simulink library "DC_GRIDSIM_LIB"  (R2022b)
settings: Solver=VariableStepAuto  StartTime=0.0  StopTime=10.0  RelTol=1e-3
undefined symbols (not defined in the file): Allday_timevector, DiscIntNeverNeededParam, High, Household1_Autumnallday, Household1_Springallday, Household1_Summerallday, Household1_Winterallday, Household9_Autumnallday, Household9_Springallday, Household9_Summerallday, Household9_Winterallday, Low, MV, Shift
libraries: fl_lib x66, nesl_utility x33, simulink x8, ee_lib x4
(part 1 of 2)
settings Model: Creator=cfn2169  LastModifiedBy=cfn2169

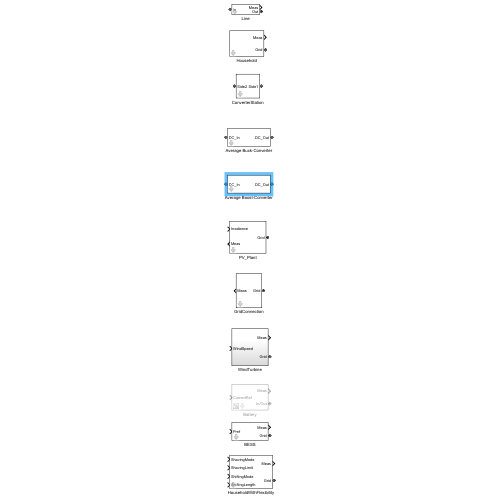
[thumbnail: Simulink's stored preview of the top-level diagram]
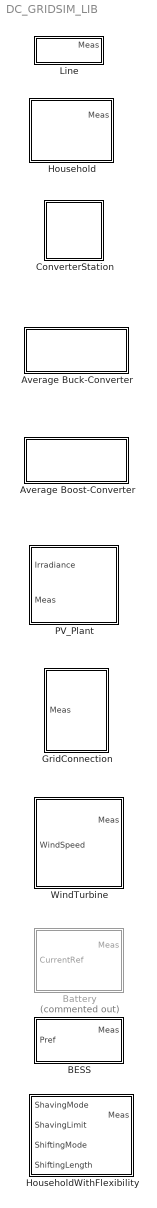
== system DC_GRIDSIM_LIB ==
  Average Boost-Converter : Subsystem  mask{C=1000, D=0.5}
      mask prompts: C "Input/Output Capacities in uF"; D "Duty Cycle"
  Average Buck-Converter : Subsystem  mask{C=1000, D=0.5}
      mask prompts: C "Input/Ouput Capacities in uF"; D "Duty Cycle"
  BESS : Subsystem  mask{V_Bat=380, Qbat=10000, SOC_init=0.5, SOC_min=0.1, SOC_max=0.9, P_max=10000}
      mask prompts: V_Bat "Nominal voltage of battery in V"; Qbat "Battery capacity in Ah"; SOC_init "Initial SOC"; SOC_min "Lower limit for SOC"; SOC_max "Upper limit for SOC"; P_max "Maximum charging/discharging power in W"
  Battery : Subsystem  Commented=on  mask{SOC_Init=0.5, Npar=5, Nser=13, Efull=4.15, Qrat=1.0, Irat=0.2, Eexp=3.7, Qexp=0.85, Enom=3.63, Qnom=0.92, Rint=0.09}
      mask prompts: SOC_Init "Initial SOC"; Npar "Number of cells in parallel"; Nser "Number of cells in series"; Efull "Fully charged voltage in V"; Qrat "Rated capacity in Ah"; Irat "Rated current in A"; Eexp "Voltage at end of exponential zone in V"; Qexp "Charge at end of exponential zone in Ah"; Enom "Voltage at end of nominal zone in V"; Qnom "Charge at end of nominal zone in Ah"; Rint "Internal resistance in Ohm"
      mask DialogControl ParameterGroupVar_1 Prompt: Stack Parameters
      mask DialogControl DescTextVar_1 Prompt: This section defines general parameters for the whole battery. The numbers of connected cells define the overall battery voltage as Vbat = Ecell*Nser and the battery capacity as Qbat = Qcell*Npar.
      mask DialogControl ParameterGroupVar_2 Prompt: Cell Parameters
      mask DialogControl DescTextVar_2 Prompt: This section defines the cell parameters for the battery. They can be found in the datasheet or can be taken from typical charging curves.
  ConverterStation : Subsystem  mask{V_Ref=380}
      mask prompts: V_Ref "Nominal voltage of secondary side"
      mask DialogControl DescTextVar Prompt: Model of a MVDC/LVDC converter station
  GridConnection : Subsystem  mask{MV_Ref=10000}
      mask prompts: MV_Ref "MV voltage reference"
  Household : Subsystem  mask{ProfileSpring=Household1_Springallday, ProfileSummer=Household1_Summerallday, ProfileAutumn=Household1_Autumnallday, ProfileWinter=Household1_Winterallday, Timevector=Allday_timevector, k=1, VnomLoad=380}
      mask prompts: ProfileSpring "Load profile for spring"; ProfileSummer "Load profile for summer"; ProfileAutumn "Load profile for autumn"; ProfileWinter "Load profile for winter"; Timevector "Corresponding timevector"; k "Scaling factor"; VnomLoad "Nominal voltage load"
      mask DialogControl DescTextVar Prompt: Profile-based load model for households
  HouseholdWithFlexibility : Subsystem  mask{Profile_spring=Household9_Springallday, Profile_summer=Household9_Summerallday, Profile_autumn=Household9_Autumnallday, Profile_winter=Household9_Winterallday, Timevector=Allday_timevector, k=1, Vload=380, Base=500, flxQuota=0.5}
      mask prompts: Profile_spring "Load profile for spring"; Profile_summer "Load profile for summer"; Profile_autumn "Load profile for autumn"; Profile_winter "Load profile for winter"; Timevector "Corresponding timevector"; k "Scaling factor"; Vload "Nominal voltage load in V"; Base "Base load in W"; flxQuota "Quota of flexible load"
  Line : Subsystem  mask{rho=1.68e-8, l=1.0, A=240e-6}
      mask prompts: rho "Specific resistivity in Ohm*m"; l "Length in m"; A "Cross sectional area in m^2"
      mask DialogControl DescTextVar Prompt: Resistive line model for two-wired DC systems
  PV_Plant : Subsystem  mask{eta_pv=0.2, area_pv=1000}
      mask prompts: eta_pv "Efficiency of PV modules"; area_pv "Effective area of PV modules in m^2"
      settings: PortSchema="{\"entries\":[{\"content\":{\"sides\":[{\"content\":{\"connectorIds\":[\"LConn1\"]},\"type\":\"ConnectorPlacement.EquallySpacedRectSide\",\"uuid\":\"e7d30e91-d877-4849-85d5-5068117b5a73\"},{\"content\":{\"connectorIds\":[\"In1\",\"Out1\"],\"side\":\"RIGHT\"},\"type\":\"ConnectorPlacement.EquallySpacedRectSide\",\"uuid\":\"aff2ec47-1e97-401e-aec0-02d86814fbc3\"},{\"content\":{\"connectorIds\":[],\"side\":\"TOP\"},\"type\":\"ConnectorPlacement.EquallySpacedRectSide\",\"uuid\":\"0abfbb66-97f7-400f-9c84-fe1e10d1a17f\"}]},\"type\":\"ConnectorPlacement.EquallySpacedConnector\",\"uuid\":\"740b86aa-7ace-499a-bee9-62f02e790000\"}],\"packageUris\":[\"http://schema.mathworks.com/mf0/Connector/R2020b\"],\"version\":\"1.0\"}"
  WindTurbine : Subsystem

== system DC_GRIDSIM_LIB/Average Boost-Converter ==
  PS Constant7 : fl_lib/Physical Signals/Sources/PS Constant  constant=D
  Resistor12 : fl_lib/Electrical/Electrical Elements/Resistor  R=1e6 Ohm  i_specify=off  i_priority=None  i=0 A  i_nominal_specify=off  i_nominal_unit=A  i_nominal_value=1  v_specify=off  v_priority=None  v=0 V  v_nominal_specify=off  v_nominal_unit=V  v_nominal_value=1
  Resistor39 : fl_lib/Electrical/Electrical Elements/Resistor  R=1e6 Ohm  i_specify=off  i_priority=None  i=0 A  i_nominal_specify=off  i_nominal_unit=A  i_nominal_value=1  v_specify=off  v_priority=None  v=0 V  v_nominal_specify=off  v_nominal_unit=V  v_nominal_value=1
  Simscape Bus1 : SimscapeBus  HierarchyStrings=High;Low
  Simscape Bus2 : SimscapeBus  HierarchyStrings=High;Low
  Subsystem5 : Subsystem
  DC_In : PMIOPort  Side=Left
  DC_Out : PMIOPort  Port=2  Side=Right
  connections:
  Resistor12/LConn1 -- Resistor39/RConn1 -- Simscape Bus1/LConn1 -- Subsystem5/RConn1
  Simscape Bus1/LConn2 -- Subsystem5/RConn2 -- Resistor12/RConn1
  Simscape Bus2/LConn2 -- Subsystem5/LConn3 -- Resistor39/LConn1
  Simscape Bus2/RConn1 -- DC_In/RConn1
  Simscape Bus1/RConn1 -- DC_Out/RConn1
  PS Constant7/RConn1 -- Subsystem5/LConn1
  Simscape Bus2/LConn1 -- Subsystem5/LConn2

== system DC_GRIDSIM_LIB/Average Buck-Converter ==
  PS Constant7 : fl_lib/Physical Signals/Sources/PS Constant  constant=D
  Resistor12 : fl_lib/Electrical/Electrical Elements/Resistor  R=1e6 Ohm  i_specify=off  i_priority=None  i=0 A  i_nominal_specify=off  i_nominal_unit=A  i_nominal_value=1  v_specify=off  v_priority=None  v=0 V  v_nominal_specify=off  v_nominal_unit=V  v_nominal_value=1
  Resistor39 : fl_lib/Electrical/Electrical Elements/Resistor  R=1e6 Ohm  i_specify=off  i_priority=None  i=0 A  i_nominal_specify=off  i_nominal_unit=A  i_nominal_value=1  v_specify=off  v_priority=None  v=0 V  v_nominal_specify=off  v_nominal_unit=V  v_nominal_value=1
  Simscape Bus1 : SimscapeBus  HierarchyStrings=High;Low
  Simscape Bus2 : SimscapeBus  HierarchyStrings=High;Low
  Subsystem5 : Subsystem
  DC_In : PMIOPort  Side=Left
  DC_Out : PMIOPort  Port=2  Side=Right
  connections:
  Subsystem5/RConn2 -- Resistor12/RConn1 -- Simscape Bus1/LConn2
  Resistor39/LConn1 -- Subsystem5/LConn3 -- Simscape Bus2/LConn2
  Resistor12/LConn1 -- Resistor39/RConn1 -- Simscape Bus1/LConn1 -- Subsystem5/RConn1
  Simscape Bus2/RConn1 -- DC_In/RConn1
  Subsystem5/LConn2 -- Simscape Bus2/LConn1
  Simscape Bus1/RConn1 -- DC_Out/RConn1
  PS Constant7/RConn1 -- Subsystem5/LConn1

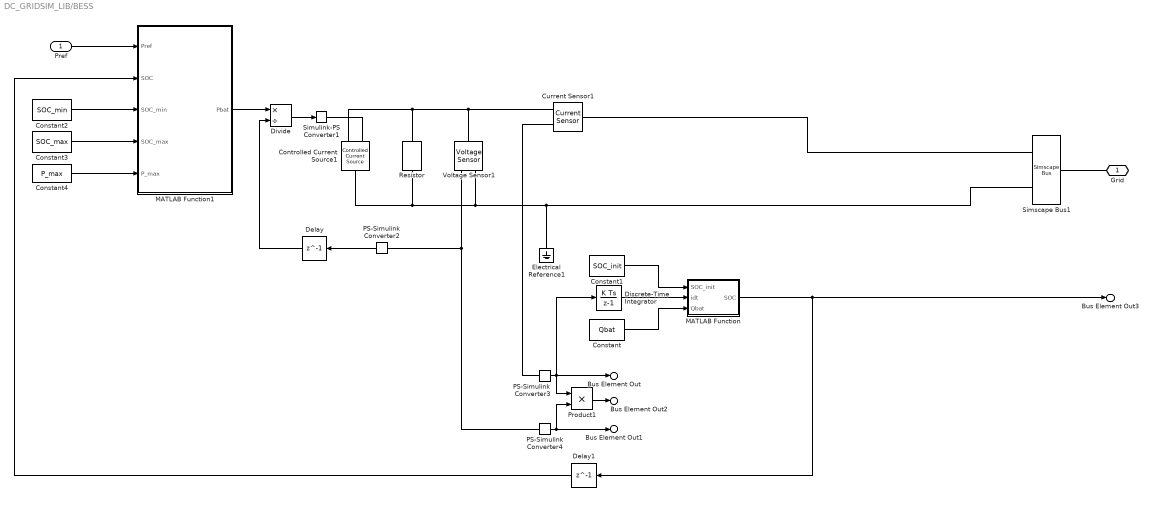
== system DC_GRIDSIM_LIB/BESS ==
  Pref : Inport
  Constant : Constant  Value=Qbat
  Constant1 : Constant  Value=SOC_init
  Constant2 : Constant  Value=SOC_min
  Constant3 : Constant  Value=SOC_max
  Constant4 : Constant  Value=P_max
  Controlled Current Source1 : fl_lib/Electrical/Electrical Sources/Controlled Current Source
  Current Sensor1 : fl_lib/Electrical/Electrical Sensors/Current Sensor
  Delay : Delay  DelayLength=1  InitialCondition=V_Bat
  Delay1 : Delay  DelayLength=1  InitialCondition=SOC_init
  Discrete-Time Integrator : DiscreteIntegrator  SampleTime=-1  ICPrevOutput=DiscIntNeverNeededParam  ICPrevScaledInput=DiscIntNeverNeededParam
  Divide : Product  Inputs=*/
  Electrical Reference1 : fl_lib/Electrical/Electrical Elements/Electrical Reference
  MATLAB Function : MATLAB Function  TreatAsAtomicUnit=on
  MATLAB Function1 : MATLAB Function  TreatAsAtomicUnit=on
  PS-Simulink Converter2 : nesl_utility/PS-Simulink Converter  PhysicalDomain=network_engine_domain  SubClassName=ps_output  LeftPortType=input  RightPortType=output  PseudoPeriodic=off  Frequencies=[]  VectorFormat=inherit  Unit=inherit  AffineConversion=off
  PS-Simulink Converter3 : nesl_utility/PS-Simulink Converter  PhysicalDomain=network_engine_domain  SubClassName=ps_output  LeftPortType=input  RightPortType=output  PseudoPeriodic=off  Frequencies=[]  VectorFormat=inherit  Unit=inherit  AffineConversion=off
  PS-Simulink Converter4 : nesl_utility/PS-Simulink Converter  PhysicalDomain=network_engine_domain  SubClassName=ps_output  LeftPortType=input  RightPortType=output  PseudoPeriodic=off  Frequencies=[]  VectorFormat=inherit  Unit=inherit  AffineConversion=off
  Product1 : Product
  Resistor : fl_lib/Electrical/Electrical Elements/Resistor  R=1e9 Ohm  i_specify=off  i_priority=None  i=0 A  i_nominal_specify=off  i_nominal_unit=A  i_nominal_value=1  v_specify=off  v_priority=None  v=0 V  v_nominal_specify=off  v_nominal_unit=V  v_nominal_value=1
  Simscape Bus1 : SimscapeBus  HierarchyStrings=High;Low
  Simulink-PS Converter1 : nesl_utility/Simulink-PS Converter  PhysicalDomain=network_engine_domain  SubClassName=ps_input  LeftPortType=input  RightPortType=output  PseudoPeriodic=off  Frequencies=[]  NoiseDistribution=none  NoiseParameters=[]  Unit=1  AffineConversion=off  FilteringAndDerivatives=provide  SimscapeFilterOrder=1  InputFilterTimeConstant=0.001  UdotUserProvided=0
  Voltage Sensor1 : fl_lib/Electrical/Electrical Sensors/Voltage Sensor
  Grid : PMIOPort  Side=Right
  Bus Element Out : Outport  PortName=Meas  Element=Current
  Bus Element Out1 : Outport  PortName=Meas  Element=Voltage
  Bus Element Out2 : Outport  PortName=Meas  Element=Power
  Bus Element Out3 : Outport  PortName=Meas  Element=SOC
  wires:
  Product1/1 -> Bus Element Out2/1
  MATLAB Function1/1(Pbat) -> Divide/1
  PS-Simulink Converter3/1 -> Discrete-Time Integrator/1, Product1/1, Bus Element Out/1
  Delay/1 -> Divide/2
  Divide/1 -> Simulink-PS Converter1/1
  PS-Simulink Converter4/1 -> Product1/2, Bus Element Out1/1
  PS-Simulink Converter2/1 -> Delay/1
  Discrete-Time Integrator/1 -> MATLAB Function/2(idt)
  Constant/1 -> MATLAB Function/3(Qbat)
  Constant1/1 -> MATLAB Function/1(SOC_init)
  MATLAB Function/1(SOC) -> Bus Element Out3/1, Delay1/1
  Pref/1 -> MATLAB Function1/1(Pref)
  Delay1/1 -> MATLAB Function1/2(SOC)
  Constant2/1 -> MATLAB Function1/3(SOC_min)
  Constant3/1 -> MATLAB Function1/4(SOC_max)
  Constant4/1 -> MATLAB Function1/5(P_max)
  connections:
  Voltage Sensor1/LConn1 -- Resistor/LConn1 -- Controlled Current Source1/RConn2 -- Current Sensor1/RConn2
  PS-Simulink Converter2/LConn1 -- PS-Simulink Converter4/LConn1 -- Voltage Sensor1/RConn1
  Simscape Bus1/LConn1 -- Current Sensor1/LConn1
  PS-Simulink Converter3/LConn1 -- Current Sensor1/RConn1
  Simulink-PS Converter1/RConn1 -- Controlled Current Source1/RConn1
  Grid/RConn1 -- Simscape Bus1/RConn1
  Resistor/RConn1 -- Controlled Current Source1/LConn1 -- Voltage Sensor1/RConn2 -- Simscape Bus1/LConn2 -- Electrical Reference1/LConn1

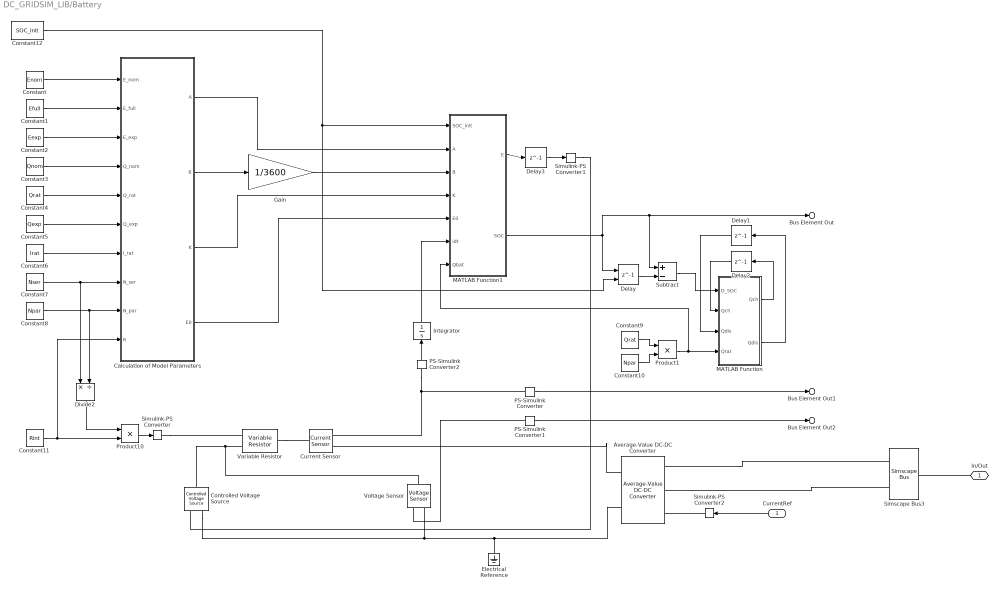
== system DC_GRIDSIM_LIB/Battery ==
  CurrentRef : Inport
  Average-Value DC-DC Converter : ee_lib/Semiconductors & Converters/Converters/Average-Value DC-DC Converter  control_option=ee.enum.converters.controlinput.current  converter_type=ee.enum.converters.dcdctype.buck  efficiency_option=ee.enum.converters.efficiency.constant  efficiency_fixed=100  i_vec=[0, 2, 5] A  efficiency_vec=[90, 95, 98]
      settings: InternalSimscapePortConfiguration="{\"Bottom\":[],\"Left\":[{\"id\":\"Iref\",\"label\":\"Iref\",\"type\":\"input\"},{\"id\":\"p1\",\"label\":\"1+\",\"type\":\"foundation.electrical.electrical\"},{\"id\":\"n1\",\"label\":\"1-\",\"type\":\"foundation.electrical.electrical\"}],\"Right\":[{\"id\":\"p2\",\"label\":\"2+\",\"type\":\"foundation.electrical.electrical\"},{\"id\":\"n2\",\"label\":\"2-\",\"type\":\"foundation.electrical.electrical\"}],\"Top\":[]}"
  Calculation of Model Parameters : Subsystem
  Constant : Constant  Value=Enom
  Constant1 : Constant  Value=Efull
  Constant10 : Constant  Value=Npar
  Constant11 : Constant  Value=Rint
  Constant12 : Constant  Value=SOC_Init
  Constant2 : Constant  Value=Eexp
  Constant3 : Constant  Value=Qnom
  Constant4 : Constant  Value=Qrat
  Constant5 : Constant  Value=Qexp
  Constant6 : Constant  Value=Irat
  Constant7 : Constant  Value=Nser
  Constant8 : Constant  Value=Npar
  Constant9 : Constant  Value=Qrat
  Controlled Voltage Source : fl_lib/Electrical/Electrical Sources/Controlled Voltage Source
  Current Sensor : fl_lib/Electrical/Electrical Sensors/Current Sensor
  Delay : Delay  DelayLength=1  InitialConditionSource=Input port
      settings: InputPortMap=u0,p4
  Delay1 : Delay  DelayLength=1
  Delay2 : Delay  DelayLength=1
  Delay3 : Delay  DelayLength=1  InitialCondition=Enom*Nser
  Divide2 : Product  Inputs=*/
  Electrical Reference : fl_lib/Electrical/Electrical Elements/Electrical Reference
  Gain : Gain  Gain=1/3600
  Integrator : Integrator
  MATLAB Function : MATLAB Function  TreatAsAtomicUnit=on
  MATLAB Function1 : MATLAB Function  TreatAsAtomicUnit=on
  PS-Simulink Converter : nesl_utility/PS-Simulink Converter  PhysicalDomain=network_engine_domain  SubClassName=ps_output  LeftPortType=input  RightPortType=output  PseudoPeriodic=off  Frequencies=[]  VectorFormat=1-D array  Unit=inherit  AffineConversion=off
  PS-Simulink Converter1 : nesl_utility/PS-Simulink Converter  PhysicalDomain=network_engine_domain  SubClassName=ps_output  LeftPortType=input  RightPortType=output  PseudoPeriodic=off  Frequencies=[]  VectorFormat=1-D array  Unit=inherit  AffineConversion=off
  PS-Simulink Converter2 : nesl_utility/PS-Simulink Converter  PhysicalDomain=network_engine_domain  SubClassName=ps_output  LeftPortType=input  RightPortType=output  PseudoPeriodic=off  Frequencies=[]  VectorFormat=1-D array  Unit=inherit  AffineConversion=off
  Product1 : Product
  Product10 : Product
  Simscape Bus3 : SimscapeBus  HierarchyStrings=Low;High
  Simulink-PS Converter : nesl_utility/Simulink-PS Converter  PhysicalDomain=network_engine_domain  SubClassName=ps_input  LeftPortType=input  RightPortType=output  PseudoPeriodic=off  Frequencies=[]  NoiseDistribution=none  NoiseParameters=[]  Unit=1  AffineConversion=off  FilteringAndDerivatives=provide  SimscapeFilterOrder=1  InputFilterTimeConstant=0.001  UdotUserProvided=0
  Simulink-PS Converter1 : nesl_utility/Simulink-PS Converter  PhysicalDomain=network_engine_domain  SubClassName=ps_input  LeftPortType=input  RightPortType=output  PseudoPeriodic=off  Frequencies=[]  NoiseDistribution=none  NoiseParameters=[]  Unit=1  AffineConversion=off  FilteringAndDerivatives=provide  SimscapeFilterOrder=1  InputFilterTimeConstant=0.001  UdotUserProvided=0
  Simulink-PS Converter2 : nesl_utility/Simulink-PS Converter  PhysicalDomain=network_engine_domain  SubClassName=ps_input  LeftPortType=input  RightPortType=output  PseudoPeriodic=off  Frequencies=[]  NoiseDistribution=none  NoiseParameters=[]  Unit=1  AffineConversion=off  FilteringAndDerivatives=provide  SimscapeFilterOrder=1  InputFilterTimeConstant=0.001  UdotUserProvided=0
  Subtract : Sum  Inputs=+-
  Variable Resistor : fl_lib/Electrical/Electrical Elements/Variable Resistor  Rmin=0 Ohm  i_specify=off  i_priority=None  i=0 A  i_nominal_specify=off  i_nominal_unit=A  i_nominal_value=1  v_specify=off  v_priority=None  v=0 V  v_nominal_specify=off  v_nominal_unit=V  v_nominal_value=1
  Voltage Sensor : fl_lib/Electrical/Electrical Sensors/Voltage Sensor
  In/Out : PMIOPort  Side=Right
  Bus Element Out : Outport  PortName=Meas  Element=SOC
  Bus Element Out1 : Outport  PortName=Meas  Element=Current
  Bus Element Out2 : Outport  PortName=Meas  Element=Voltage
  wires:
  Integrator/1 -> MATLAB Function1/6(idt)
  Constant7/1 -> Calculation of Model Parameters/8(N_ser), Divide2/1
  MATLAB Function/2(Qdis) -> Delay1/1
  PS-Simulink Converter2/1 -> Integrator/1
  Constant8/1 -> Calculation of Model Parameters/9(N_par), Divide2/2
  Calculation of Model Parameters/3(K) -> MATLAB Function1/4(K)
  Delay2/1 -> MATLAB Function/2("Qch ")
  MATLAB Function/1(Qch) -> Delay2/1
  Constant9/1 -> Product1/1
  PS-Simulink Converter1/1 -> Bus Element Out2/1
  PS-Simulink Converter/1 -> Bus Element Out1/1
  Calculation of Model Parameters/4(E0) -> MATLAB Function1/5(E0)
  Delay1/1 -> MATLAB Function/3("Qdis ")
  Gain/1 -> MATLAB Function1/3(B)
  Calculation of Model Parameters/1(A) -> MATLAB Function1/2(A)
  Constant12/1 -> Delay/2, MATLAB Function1/1(SOC_init)
  Product10/1 -> Simulink-PS Converter/1
  Constant/1 -> Calculation of Model Parameters/1(E_nom)
  Calculation of Model Parameters/2(B) -> Gain/1
  Constant1/1 -> Calculation of Model Parameters/2(E_full)
  Subtract/1 -> MATLAB Function/1(D_SOC)
  Constant6/1 -> Calculation of Model Parameters/7(I_rat)
  Constant10/1 -> Product1/2
  Constant4/1 -> Calculation of Model Parameters/5(Q_rat)
  Constant5/1 -> Calculation of Model Parameters/6(Q_exp)
  Divide2/1 -> Product10/1
  MATLAB Function1/2(SOC) -> Bus Element Out/1, Subtract/1, Delay/1
  Constant11/1 -> Product10/2, Calculation of Model Parameters/10(R)
  Constant3/1 -> Calculation of Model Parameters/4(Q_nom)
  Constant2/1 -> Calculation of Model Parameters/3(E_exp)
  Product1/1 -> MATLAB Function1/7(Qbat), MATLAB Function/4(Qrat)
  Delay/1 -> Subtract/2
  MATLAB Function1/1(E) -> Delay3/1
  Delay3/1 -> Simulink-PS Converter1/1
  CurrentRef/1 -> Simulink-PS Converter2/1
  connections:
  PS-Simulink Converter/LConn1 -- PS-Simulink Converter2/LConn1 -- Current Sensor/RConn1
  Electrical Reference/LConn1 -- Average-Value DC-DC Converter/RConn1 -- Controlled Voltage Source/RConn2 -- Voltage Sensor/RConn2
  Voltage Sensor/LConn1 -- Controlled Voltage Source/LConn1 -- Variable Resistor/LConn2
  Simulink-PS Converter1/RConn1 -- Controlled Voltage Source/RConn1
  Average-Value DC-DC Converter/RConn2 -- Current Sensor/RConn2
  Simulink-PS Converter/RConn1 -- Variable Resistor/LConn1
  Variable Resistor/RConn1 -- Current Sensor/LConn1
  PS-Simulink Converter1/LConn1 -- Voltage Sensor/RConn1
  Simulink-PS Converter2/RConn1 -- Average-Value DC-DC Converter/LConn1
  In/Out/RConn1 -- Simscape Bus3/RConn1
  Simscape Bus3/LConn2 -- Average-Value DC-DC Converter/LConn2
  Simscape Bus3/LConn1 -- Average-Value DC-DC Converter/LConn3

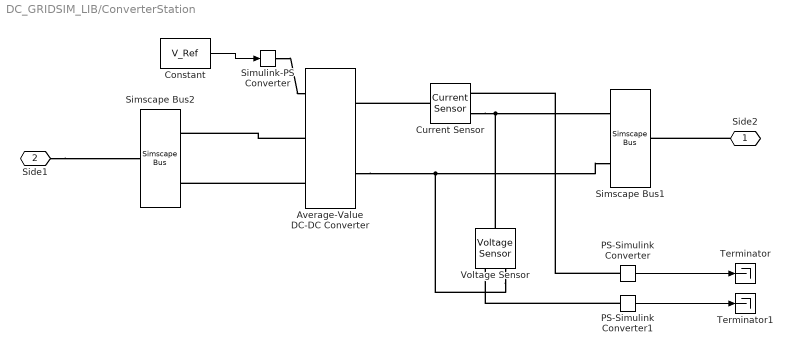
== system DC_GRIDSIM_LIB/ConverterStation ==
  Average-Value DC-DC Converter : ee_lib/Semiconductors & Converters/Converters/Average-Value DC-DC Converter  control_option=ee.enum.converters.controlinput.voltage  converter_type=ee.enum.converters.dcdctype.buck  efficiency_option=ee.enum.converters.efficiency.constant  efficiency_fixed=100  i_vec=[0, 2, 5] A  efficiency_vec=[90, 95, 98]
      settings: InternalSimscapePortConfiguration="{\"Bottom\":[],\"Left\":[{\"id\":\"Vref\",\"label\":\"Vref\",\"type\":\"input\"},{\"id\":\"p1\",\"label\":\"1+\",\"type\":\"foundation.electrical.electrical\"},{\"id\":\"n1\",\"label\":\"1-\",\"type\":\"foundation.electrical.electrical\"}],\"Right\":[{\"id\":\"p2\",\"label\":\"2+\",\"type\":\"foundation.electrical.electrical\"},{\"id\":\"n2\",\"label\":\"2-\",\"type\":\"foundation.electrical.electrical\"}],\"Top\":[]}"
  Constant : Constant  Value=V_Ref
  Current Sensor : fl_lib/Electrical/Electrical Sensors/Current Sensor
  PS-Simulink Converter : nesl_utility/PS-Simulink Converter  PhysicalDomain=network_engine_domain  SubClassName=ps_output  LeftPortType=input  RightPortType=output  PseudoPeriodic=off  Frequencies=[]  VectorFormat=inherit  Unit=inherit  AffineConversion=off
  PS-Simulink Converter1 : nesl_utility/PS-Simulink Converter  PhysicalDomain=network_engine_domain  SubClassName=ps_output  LeftPortType=input  RightPortType=output  PseudoPeriodic=off  Frequencies=[]  VectorFormat=inherit  Unit=inherit  AffineConversion=off
  Simscape Bus1 : SimscapeBus  HierarchyStrings=High;Low
  Simscape Bus2 : SimscapeBus  HierarchyStrings=High;Low
  Simulink-PS Converter : nesl_utility/Simulink-PS Converter  PhysicalDomain=network_engine_domain  SubClassName=ps_input  LeftPortType=input  RightPortType=output  PseudoPeriodic=off  Frequencies=[]  NoiseDistribution=none  NoiseParameters=[]  Unit=1  AffineConversion=off  FilteringAndDerivatives=provide  SimscapeFilterOrder=1  InputFilterTimeConstant=0.001  UdotUserProvided=0
  Terminator : Terminator
  Terminator1 : Terminator
  Voltage Sensor : fl_lib/Electrical/Electrical Sensors/Voltage Sensor
  Side2 : PMIOPort  Side=Left
  Side1 : PMIOPort  Port=2  Side=Right
  wires:
  PS-Simulink Converter/1 -> Terminator/1
  PS-Simulink Converter1/1 -> Terminator1/1
  Constant/1 -> Simulink-PS Converter/1
  connections:
  Voltage Sensor/RConn2 -- Average-Value DC-DC Converter/RConn2 -- Simscape Bus1/LConn2
  Voltage Sensor/LConn1 -- Simscape Bus1/LConn1 -- Current Sensor/RConn2
  Current Sensor/LConn1 -- Average-Value DC-DC Converter/RConn1
  PS-Simulink Converter/LConn1 -- Current Sensor/RConn1
  Average-Value DC-DC Converter/LConn2 -- Simscape Bus2/LConn1
  Average-Value DC-DC Converter/LConn3 -- Simscape Bus2/LConn2
  Simulink-PS Converter/RConn1 -- Average-Value DC-DC Converter/LConn1
  PS-Simulink Converter1/LConn1 -- Voltage Sensor/RConn1
  Side2/RConn1 -- Simscape Bus1/RConn1
  Side1/RConn1 -- Simscape Bus2/RConn1

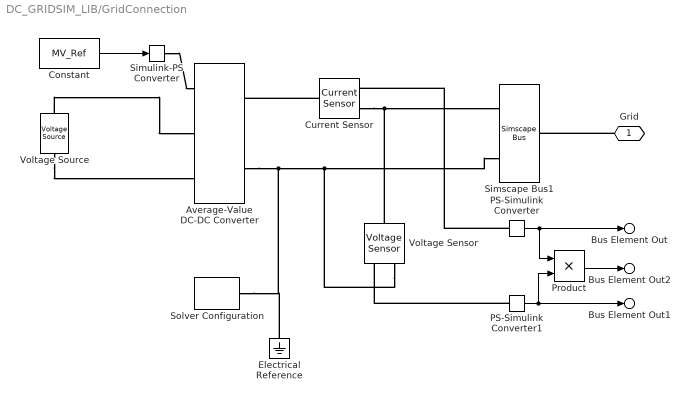
== system DC_GRIDSIM_LIB/GridConnection ==
  Average-Value DC-DC Converter : ee_lib/Semiconductors & Converters/Converters/Average-Value DC-DC Converter  control_option=ee.enum.converters.controlinput.voltage  converter_type=ee.enum.converters.dcdctype.buck  efficiency_option=ee.enum.converters.efficiency.constant  efficiency_fixed=100  i_vec=[0, 2, 5] A  efficiency_vec=[90, 95, 98]
      settings: InternalSimscapePortConfiguration="{\"Bottom\":[],\"Left\":[{\"id\":\"Vref\",\"label\":\"Vref\",\"type\":\"input\"},{\"id\":\"p1\",\"label\":\"1+\",\"type\":\"foundation.electrical.electrical\"},{\"id\":\"n1\",\"label\":\"1-\",\"type\":\"foundation.electrical.electrical\"}],\"Right\":[{\"id\":\"p2\",\"label\":\"2+\",\"type\":\"foundation.electrical.electrical\"},{\"id\":\"n2\",\"label\":\"2-\",\"type\":\"foundation.electrical.electrical\"}],\"Top\":[]}"
  Constant : Constant  Value=MV_Ref
  Current Sensor : fl_lib/Electrical/Electrical Sensors/Current Sensor
  Electrical Reference : fl_lib/Electrical/Electrical Elements/Electrical Reference
  PS-Simulink Converter : nesl_utility/PS-Simulink Converter  PhysicalDomain=network_engine_domain  SubClassName=ps_output  LeftPortType=input  RightPortType=output  PseudoPeriodic=off  Frequencies=[]  VectorFormat=inherit  Unit=inherit  AffineConversion=off
  PS-Simulink Converter1 : nesl_utility/PS-Simulink Converter  PhysicalDomain=network_engine_domain  SubClassName=ps_output  LeftPortType=input  RightPortType=output  PseudoPeriodic=off  Frequencies=[]  VectorFormat=inherit  Unit=inherit  AffineConversion=off
  Product : Product
  Simscape Bus1 : SimscapeBus  HierarchyStrings=High;Low
  Simulink-PS Converter : nesl_utility/Simulink-PS Converter  PhysicalDomain=network_engine_domain  SubClassName=ps_input  LeftPortType=input  RightPortType=output  PseudoPeriodic=off  Frequencies=[]  NoiseDistribution=none  NoiseParameters=[]  Unit=1  AffineConversion=off  FilteringAndDerivatives=provide  SimscapeFilterOrder=1  InputFilterTimeConstant=0.001  UdotUserProvided=0
  Solver Configuration : nesl_utility/Solver Configuration  PhysicalDomain=network_engine_domain  SubClassName=solver  LeftPortType=input  RightPortType=generic  Tones=[]  Harmonics=[]  SimulateNoise=off  Profile=off  UseLocalSampling=off  EnableSwitchedLinearOptims=on  FrequencyDomain=off  UseCCode=off  RelTol=0.001  AbsTol=0.001  MinStep=1e-09  ToWorkspace=off  RevertToSquareIcSolve=off  NumHomotopyIterations=100  PhasorMode=off  PhasorModeNumHarmonics=1  ConsistencySolver=NEWTON_XTOL_AFTER_FTOL  IndexReductionMethod=DerivativeReplacement  DoDC=off  ResidualTolerance=1e-09  ConsistencyTolSource=GLOBAL  ConsistencyAbsTol=0.001  ConsistencyRelTol=0.001  ConsistencyTolFactor=0.001  UseLocalSolver=off  LocalSolverChoice=NE_BACKWARD_EULER_ADVANCER  ResolveIndetEquations=on  FunctionEvalNumThread=1  LocalSolverSampleTime=0.001  DoFixedCost=off  MaxNonlinIter=3  MaxModeIter=2  ComputeImpulses=off  ImpulseIterations=2  LinearAlgebra=auto  LinearAlgebraNumThread=0  EquationFormulation=NE_TIME_EF  DelaysMemoryBudget=1024  AutomaticFiltering=on  FilteringTimeConstant=0.001  PartitionStorageMethod=AS_NEEDED  PartitionMemoryBudget=1024  PartitionMethod=ROBUST
  Voltage Sensor : fl_lib/Electrical/Electrical Sensors/Voltage Sensor
  Voltage Source : ee_lib/Sources/Voltage Source  dc_voltage=10000 V  ac_voltage=0 V  ac_shift=0 rad  ac_frequency=60 Hz  noise_mode=ee.enum.sources.noise.Disabled  PSD=0 V^2/Hz  sample_time=1e-3 s  repeatability=ee.enum.sources.repeatability.NotRepeatable  user_seed=0  auto_seed=3499211588  i_specify=off  i_priority=None  i=0 A  i_nominal_specify=off  i_nominal_unit=A  i_nominal_value=1  v_specify=off  v_priority=None  v=0 V  v_nominal_specify=off  v_nominal_unit=V  v_nominal_value=1
  Grid : PMIOPort  Side=Left
  Bus Element Out : Outport  PortName=Meas  Element=Current
  Bus Element Out1 : Outport  PortName=Meas  Element=Voltage
  Bus Element Out2 : Outport  PortName=Meas  Element=Power
  wires:
  Constant/1 -> Simulink-PS Converter/1
  PS-Simulink Converter/1 -> Product/1, Bus Element Out/1
  PS-Simulink Converter1/1 -> Product/2, Bus Element Out1/1
  Product/1 -> Bus Element Out2/1
  connections:
  Grid/RConn1 -- Simscape Bus1/RConn1
  Voltage Source/LConn1 -- Average-Value DC-DC Converter/LConn2
  Voltage Source/RConn1 -- Average-Value DC-DC Converter/LConn3
  Simulink-PS Converter/RConn1 -- Average-Value DC-DC Converter/LConn1
  Average-Value DC-DC Converter/RConn2 -- Solver Configuration/RConn1 -- Electrical Reference/LConn1 -- Voltage Sensor/RConn2 -- Simscape Bus1/LConn2
  Current Sensor/RConn2 -- Voltage Sensor/LConn1 -- Simscape Bus1/LConn1
  Current Sensor/LConn1 -- Average-Value DC-DC Converter/RConn1
  PS-Simulink Converter1/LConn1 -- Voltage Sensor/RConn1
  PS-Simulink Converter/LConn1 -- Current Sensor/RConn1

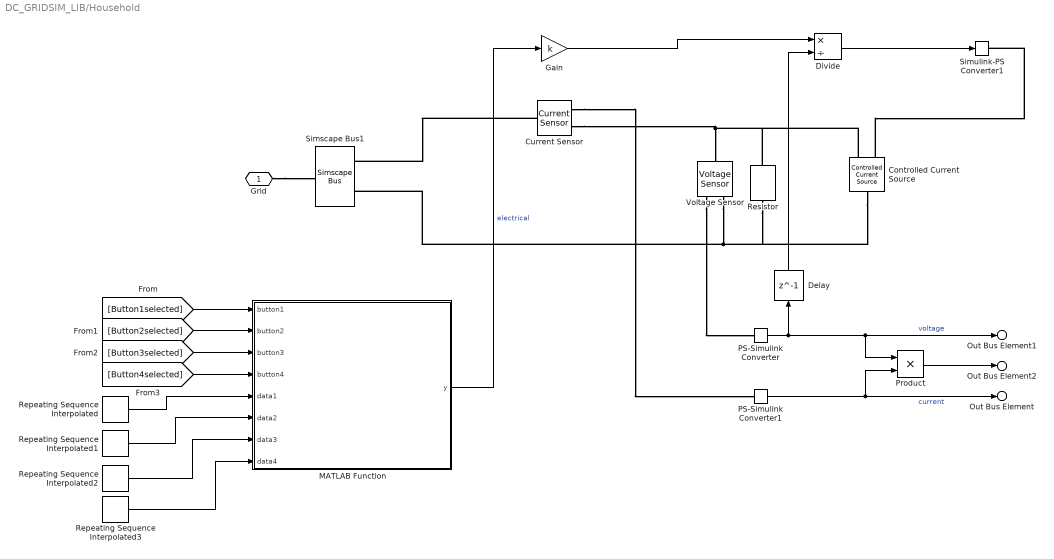
== system DC_GRIDSIM_LIB/Household ==
  Controlled Current Source : fl_lib/Electrical/Electrical Sources/Controlled Current Source
  Current Sensor : fl_lib/Electrical/Electrical Sensors/Current Sensor
  Delay : Delay  DelayLength=1  InitialCondition=VnomLoad
  Divide : Product  Inputs=*/
  Gain : Gain  Gain=k
  MATLAB Function : MATLAB Function  TreatAsAtomicUnit=on
  PS-Simulink Converter : nesl_utility/PS-Simulink Converter  PhysicalDomain=network_engine_domain  SubClassName=ps_output  LeftPortType=input  RightPortType=output  PseudoPeriodic=off  Frequencies=[]  VectorFormat=inherit  Unit=inherit  AffineConversion=off
  PS-Simulink Converter1 : nesl_utility/PS-Simulink Converter  PhysicalDomain=network_engine_domain  SubClassName=ps_output  LeftPortType=input  RightPortType=output  PseudoPeriodic=off  Frequencies=[]  VectorFormat=inherit  Unit=inherit  AffineConversion=off
  Product : Product
  Repeating Sequence Interpolated : simulink/Sources/Repeating Sequence Interpolated  OutValues=ProfileSpring  TimeValues=Timevector  LookUpMeth=Interpolation-Use End Values  tsamp=0.01  OutMin=[]  OutMax=[]  OutDataTypeStr=double  OutputDataTypeScalingMode=double  OutDataType=fixdt(0,8)  OutScaling=2^-10
  Repeating Sequence Interpolated1 : simulink/Sources/Repeating Sequence Interpolated  OutValues=ProfileSummer  TimeValues=Timevector  LookUpMeth=Interpolation-Use End Values  tsamp=0.01  OutMin=[]  OutMax=[]  OutDataTypeStr=double  OutputDataTypeScalingMode=double  OutDataType=fixdt(0,8)  OutScaling=2^-10
  Repeating Sequence Interpolated2 : simulink/Sources/Repeating Sequence Interpolated  OutValues=ProfileAutumn  TimeValues=Timevector  LookUpMeth=Interpolation-Use End Values  tsamp=0.01  OutMin=[]  OutMax=[]  OutDataTypeStr=double  OutputDataTypeScalingMode=double  OutDataType=fixdt(0,8)  OutScaling=2^-10
  Repeating Sequence Interpolated3 : simulink/Sources/Repeating Sequence Interpolated  OutValues=ProfileWinter  TimeValues=Timevector  LookUpMeth=Interpolation-Use End Values  tsamp=0.01  OutMin=[]  OutMax=[]  OutDataTypeStr=double  OutputDataTypeScalingMode=double  OutDataType=fixdt(0,8)  OutScaling=2^-10
  Resistor : fl_lib/Electrical/Electrical Elements/Resistor  R=1e9 Ohm  i_specify=off  i_priority=None  i=0 A  i_nominal_specify=off  i_nominal_unit=A  i_nominal_value=1  v_specify=off  v_priority=None  v=0 V  v_nominal_specify=off  v_nominal_unit=V  v_nominal_value=1
  Simscape Bus1 : SimscapeBus  HierarchyStrings=High;Low
  Simulink-PS Converter1 : nesl_utility/Simulink-PS Converter  PhysicalDomain=network_engine_domain  SubClassName=ps_input  LeftPortType=input  RightPortType=output  PseudoPeriodic=off  Frequencies=[]  NoiseDistribution=none  NoiseParameters=[]  Unit=1  AffineConversion=off  FilteringAndDerivatives=provide  SimscapeFilterOrder=1  InputFilterTimeConstant=0.001  UdotUserProvided=0
  Voltage Sensor : fl_lib/Electrical/Electrical Sensors/Voltage Sensor
  Grid : PMIOPort  Side=Right
  Out Bus Element : Outport  PortName=Meas  Element=Current
  Out Bus Element1 : Outport  PortName=Meas  Element=Voltage
  Out Bus Element2 : Outport  PortName=Meas  Element=Power
  wires:
  MATLAB Function/1(y) -> Gain/1  "electrical"
  PS-Simulink Converter/1 -> Delay/1, Product/1, Out Bus Element1/1  "voltage"
  PS-Simulink Converter1/1 -> Product/2, Out Bus Element/1  "current"
  [Button4selected] -> MATLAB Function/4(button4)
  [Button3selected] -> MATLAB Function/3(button3)
  [Button2selected] -> MATLAB Function/2(button2)
  [Button1selected] -> MATLAB Function/1(button1)
  Repeating Sequence Interpolated/1 -> MATLAB Function/5(data1)
  Repeating Sequence Interpolated1/1 -> MATLAB Function/6(data2)
  Repeating Sequence Interpolated2/1 -> MATLAB Function/7(data3)
  Repeating Sequence Interpolated3/1 -> MATLAB Function/8(data4)
  Product/1 -> Out Bus Element2/1
  Gain/1 -> Divide/1
  Delay/1 -> Divide/2
  Divide/1 -> Simulink-PS Converter1/1
  connections:
  Grid/RConn1 -- Simscape Bus1/RConn1
  Voltage Sensor/RConn2 -- Resistor/RConn1 -- Controlled Current Source/LConn1 -- Simscape Bus1/LConn2
  Voltage Sensor/RConn1 -- PS-Simulink Converter/LConn1
  Current Sensor/RConn1 -- PS-Simulink Converter1/LConn1
  Current Sensor/LConn1 -- Simscape Bus1/LConn1
  Current Sensor/RConn2 -- Resistor/LConn1 -- Controlled Current Source/RConn2 -- Voltage Sensor/LConn1
  Controlled Current Source/RConn1 -- Simulink-PS Converter1/RConn1

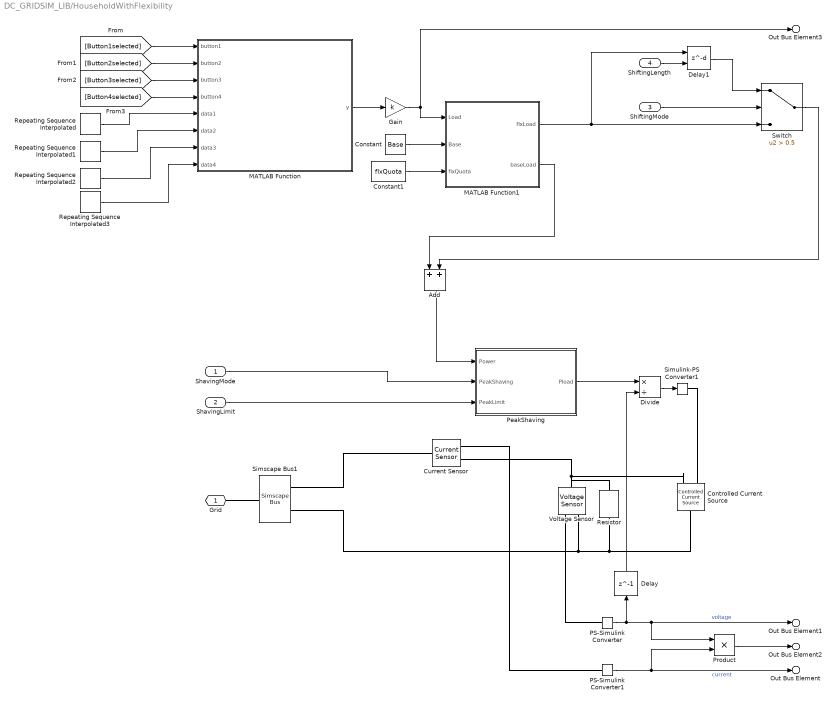
== system DC_GRIDSIM_LIB/HouseholdWithFlexibility ==
  ShavingMode : Inport
  ShavingLimit : Inport  Port=2
  ShiftingMode : Inport  Port=3
  ShiftingLength : Inport  Port=4
  Add : Sum
  Constant : Constant  Value=Base
  Constant1 : Constant  Value=flxQuota
  Controlled Current Source : fl_lib/Electrical/Electrical Sources/Controlled Current Source
  Current Sensor : fl_lib/Electrical/Electrical Sensors/Current Sensor
  Delay : Delay  DelayLength=1  InitialCondition=Vload
  Delay1 : Delay  DelayLengthSource=Input port  DelayLength=Shift  DelayLengthUpperLimit=1000
      settings: InputPortMap=u0,p1
  Divide : Product  Inputs=*/
  Gain : Gain  Gain=k
  MATLAB Function : MATLAB Function  TreatAsAtomicUnit=on
  MATLAB Function1 : MATLAB Function  TreatAsAtomicUnit=on
  PS-Simulink Converter : nesl_utility/PS-Simulink Converter  PhysicalDomain=network_engine_domain  SubClassName=ps_output  LeftPortType=input  RightPortType=output  PseudoPeriodic=off  Frequencies=[]  VectorFormat=inherit  Unit=inherit  AffineConversion=off
  PS-Simulink Converter1 : nesl_utility/PS-Simulink Converter  PhysicalDomain=network_engine_domain  SubClassName=ps_output  LeftPortType=input  RightPortType=output  PseudoPeriodic=off  Frequencies=[]  VectorFormat=inherit  Unit=inherit  AffineConversion=off
  PeakShaving : MATLAB Function  TreatAsAtomicUnit=on
  Product : Product
  Repeating Sequence Interpolated : simulink/Sources/Repeating Sequence Interpolated  OutValues=Profile_spring  TimeValues=Timevector  LookUpMeth=Interpolation-Use End Values  tsamp=0.01  OutMin=[]  OutMax=[]  OutDataTypeStr=double  OutputDataTypeScalingMode=double  OutDataType=fixdt(0,8)  OutScaling=2^-10
  Repeating Sequence Interpolated1 : simulink/Sources/Repeating Sequence Interpolated  OutValues=Profile_summer  TimeValues=Timevector  LookUpMeth=Interpolation-Use End Values  tsamp=0.01  OutMin=[]  OutMax=[]  OutDataTypeStr=double  OutputDataTypeScalingMode=double  OutDataType=fixdt(0,8)  OutScaling=2^-10
  Repeating Sequence Interpolated2 : simulink/Sources/Repeating Sequence Interpolated  OutValues=Profile_autumn  TimeValues=Timevector  LookUpMeth=Interpolation-Use End Values  tsamp=0.01  OutMin=[]  OutMax=[]  OutDataTypeStr=double  OutputDataTypeScalingMode=double  OutDataType=fixdt(0,8)  OutScaling=2^-10
  Repeating Sequence Interpolated3 : simulink/Sources/Repeating Sequence Interpolated  OutValues=Profile_winter  TimeValues=Timevector  LookUpMeth=Interpolation-Use End Values  tsamp=0.01  OutMin=[]  OutMax=[]  OutDataTypeStr=double  OutputDataTypeScalingMode=double  OutDataType=fixdt(0,8)  OutScaling=2^-10
  Resistor : fl_lib/Electrical/Electrical Elements/Resistor  R=1e9 Ohm  i_specify=off  i_priority=None  i=0 A  i_nominal_specify=off  i_nominal_unit=A  i_nominal_value=1  v_specify=off  v_priority=None  v=0 V  v_nominal_specify=off  v_nominal_unit=V  v_nominal_value=1
  Simscape Bus1 : SimscapeBus  HierarchyStrings=High;Low
  Simulink-PS Converter1 : nesl_utility/Simulink-PS Converter  PhysicalDomain=network_engine_domain  SubClassName=ps_input  LeftPortType=input  RightPortType=output  PseudoPeriodic=off  Frequencies=[]  NoiseDistribution=none  NoiseParameters=[]  Unit=A  AffineConversion=off  FilteringAndDerivatives=provide  SimscapeFilterOrder=1  InputFilterTimeConstant=0.001  UdotUserProvided=0
  Switch : Switch  Criteria=u2 > Threshold  Threshold=0.5  SaturateOnIntegerOverflow=off  InputSameDT=off
  Voltage Sensor : fl_lib/Electrical/Electrical Sensors/Voltage Sensor
  Grid : PMIOPort  Side=Right
  Out Bus Element : Outport  PortName=Meas  Element=Current
  Out Bus Element1 : Outport  PortName=Meas  Element=Voltage
  Out Bus Element2 : Outport  PortName=Meas  Element=Power
  Out Bus Element3 : Outport  PortName=Meas  Element=OriginalProfile
  wires:
  Delay/1 -> Divide/2
  Repeating Sequence Interpolated/1 -> MATLAB Function/5(data1)
  PS-Simulink Converter/1 -> Product/1, Out Bus Element1/1, Delay/1  "voltage"
  Product/1 -> Out Bus Element2/1
  Repeating Sequence Interpolated3/1 -> MATLAB Function/8(data4)
  [Button1selected] -> MATLAB Function/1(button1)
  Repeating Sequence Interpolated2/1 -> MATLAB Function/7(data3)
  Gain/1 -> MATLAB Function1/1(Load), Out Bus Element3/1
  Repeating Sequence Interpolated1/1 -> MATLAB Function/6(data2)
  Divide/1 -> Simulink-PS Converter1/1
  [Button3selected] -> MATLAB Function/3(button3)
  PS-Simulink Converter1/1 -> Product/2, Out Bus Element/1  "current"
  [Button2selected] -> MATLAB Function/2(button2)
  MATLAB Function/1(y) -> Gain/1
  [Button4selected] -> MATLAB Function/4(button4)
  PeakShaving/1(Pload) -> Divide/1
  ShavingMode/1 -> PeakShaving/2(PeakShaving)
  ShavingLimit/1 -> PeakShaving/3(PeakLimit)
  Add/1 -> PeakShaving/1(Power)
  MATLAB Function1/2(baseLoad) -> Add/1
  MATLAB Function1/1(flxLoad) -> Delay1/1, Switch/3
  Delay1/1 -> Switch/1
  ShiftingMode/1 -> Switch/2
  Switch/1 -> Add/2
  ShiftingLength/1 -> Delay1/2
  Constant/1 -> MATLAB Function1/2(Base)
  Constant1/1 -> MATLAB Function1/3(flxQuota)
  connections:
  Voltage Sensor/LConn1 -- Current Sensor/RConn2 -- Resistor/LConn1 -- Controlled Current Source/RConn2
  Simscape Bus1/LConn2 -- Voltage Sensor/RConn2 -- Resistor/RConn1 -- Controlled Current Source/LConn1
  Current Sensor/RConn1 -- PS-Simulink Converter1/LConn1
  Grid/RConn1 -- Simscape Bus1/RConn1
  Voltage Sensor/RConn1 -- PS-Simulink Converter/LConn1
  Simulink-PS Converter1/RConn1 -- Controlled Current Source/RConn1
  Current Sensor/LConn1 -- Simscape Bus1/LConn1

== system DC_GRIDSIM_LIB/Line ==
  Current Sensor : fl_lib/Electrical/Electrical Sensors/Current Sensor
  PS-Simulink Converter : nesl_utility/PS-Simulink Converter  PhysicalDomain=network_engine_domain  SubClassName=ps_output  LeftPortType=input  RightPortType=output  PseudoPeriodic=off  Frequencies=[]  VectorFormat=inherit  Unit=inherit  AffineConversion=off
  PS-Simulink Converter1 : nesl_utility/PS-Simulink Converter  PhysicalDomain=network_engine_domain  SubClassName=ps_output  LeftPortType=input  RightPortType=output  PseudoPeriodic=off  Frequencies=[]  VectorFormat=inherit  Unit=inherit  AffineConversion=off
  Resistor : fl_lib/Electrical/Electrical Elements/Resistor  R=rho*l/A Ohm  i_specify=off  i_priority=None  i=0 A  i_nominal_specify=off  i_nominal_unit=A  i_nominal_value=1  v_specify=off  v_priority=None  v=0 V  v_nominal_specify=off  v_nominal_unit=V  v_nominal_value=1
  Resistor1 : fl_lib/Electrical/Electrical Elements/Resistor  R=rho*l/A Ohm  i_specify=off  i_priority=None  i=0 A  i_nominal_specify=off  i_nominal_unit=A  i_nominal_value=1  v_specify=off  v_priority=None  v=0 V  v_nominal_specify=off  v_nominal_unit=V  v_nominal_value=1
  Simscape Bus2 : SimscapeBus  HierarchyStrings=High;Low
  Simscape Bus3 : SimscapeBus  HierarchyStrings=High;Low
  Voltage Sensor : fl_lib/Electrical/Electrical Sensors/Voltage Sensor
  In : PMIOPort  Side=Left
  Out : PMIOPort  Port=2  Side=Right
  Bus Element Out : Outport  PortName=Meas  Element=current
  Bus Element Out1 : Outport  PortName=Meas  Element=voltage
  wires:
  PS-Simulink Converter/1 -> Bus Element Out/1  "current"
  PS-Simulink Converter1/1 -> Bus Element Out1/1  "voltage"
  connections:
  Simscape Bus2/LConn1 -- Resistor/LConn1
  Simscape Bus3/LConn2 -- Voltage Sensor/RConn2 -- Resistor1/RConn1
  Simscape Bus2/RConn1 -- In/RConn1
  Resistor1/LConn1 -- Simscape Bus2/LConn2
  Simscape Bus3/RConn1 -- Out/RConn1
  Current Sensor/LConn1 -- Voltage Sensor/LConn1 -- Resistor/RConn1
  Current Sensor/RConn2 -- Simscape Bus3/LConn1
  PS-Simulink Converter/LConn1 -- Current Sensor/RConn1
  PS-Simulink Converter1/LConn1 -- Voltage Sensor/RConn1

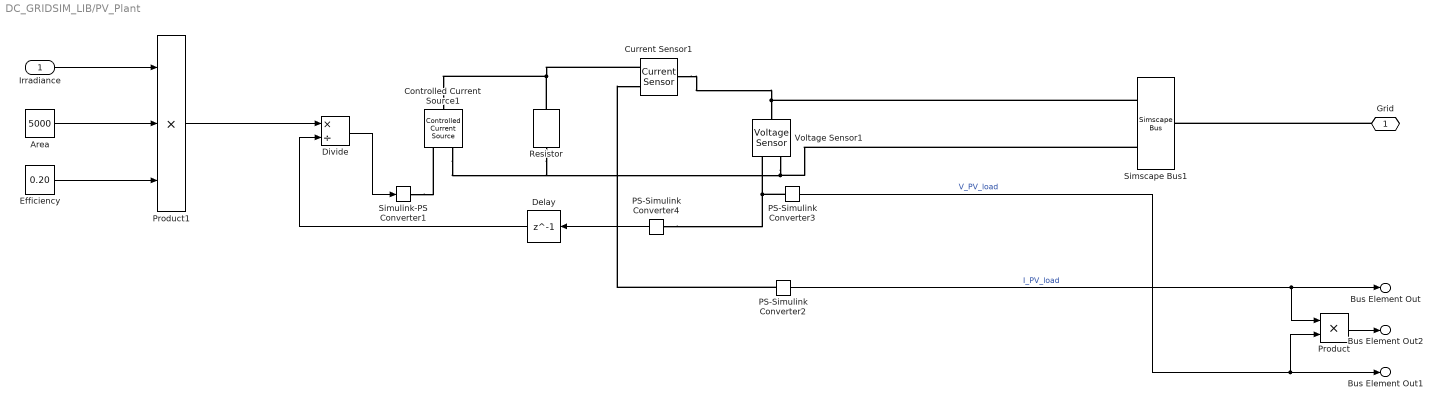
== system DC_GRIDSIM_LIB/PV_Plant ==
  Irradiance : Inport
  Area : Constant  Value=5000
  Controlled Current Source1 : fl_lib/Electrical/Electrical Sources/Controlled Current Source
  Current Sensor1 : fl_lib/Electrical/Electrical Sensors/Current Sensor
  Delay : Delay  DelayLength=1  InitialCondition=MV
  Divide : Product  Inputs=*/
  Efficiency : Constant  Value=0.20
  PS-Simulink Converter2 : nesl_utility/PS-Simulink Converter  PhysicalDomain=network_engine_domain  SubClassName=ps_output  LeftPortType=input  RightPortType=output  PseudoPeriodic=off  Frequencies=[]  VectorFormat=1-D array  Unit=inherit  AffineConversion=off
  PS-Simulink Converter3 : nesl_utility/PS-Simulink Converter  PhysicalDomain=network_engine_domain  SubClassName=ps_output  LeftPortType=input  RightPortType=output  PseudoPeriodic=off  Frequencies=[]  VectorFormat=1-D array  Unit=inherit  AffineConversion=off
  PS-Simulink Converter4 : nesl_utility/PS-Simulink Converter  PhysicalDomain=network_engine_domain  SubClassName=ps_output  LeftPortType=input  RightPortType=output  PseudoPeriodic=off  Frequencies=[]  VectorFormat=inherit  Unit=inherit  AffineConversion=off
  Product : Product
  Product1 : Product  Inputs=3
  Resistor : fl_lib/Electrical/Electrical Elements/Resistor  R=1e9 Ohm  i_specify=off  i_priority=None  i=0 A  i_nominal_specify=off  i_nominal_unit=A  i_nominal_value=1  v_specify=off  v_priority=None  v=0 V  v_nominal_specify=off  v_nominal_unit=V  v_nominal_value=1
  Simscape Bus1 : SimscapeBus  HierarchyStrings=High;Low
  Simulink-PS Converter1 : nesl_utility/Simulink-PS Converter  PhysicalDomain=network_engine_domain  SubClassName=ps_input  LeftPortType=input  RightPortType=output  PseudoPeriodic=off  Frequencies=[]  NoiseDistribution=none  NoiseParameters=[]  Unit=A  AffineConversion=off  FilteringAndDerivatives=provide  SimscapeFilterOrder=1  InputFilterTimeConstant=0.001  UdotUserProvided=0
  Voltage Sensor1 : fl_lib/Electrical/Electrical Sensors/Voltage Sensor
  Grid : PMIOPort  Side=Left
  Bus Element Out : Outport  PortName=Meas  Element=Current
  Bus Element Out1 : Outport  PortName=Meas  Element=Voltage
  Bus Element Out2 : Outport  PortName=Meas  Element=Power
  wires:
  Area/1 -> Product1/2
  Efficiency/1 -> Product1/3
  Irradiance/1 -> Product1/1
  Delay/1 -> Divide/2
  Divide/1 -> Simulink-PS Converter1/1
  PS-Simulink Converter3/1 -> Product/2, Bus Element Out1/1  "V_PV_load"
  PS-Simulink Converter4/1 -> Delay/1
  Product1/1 -> Divide/1
  PS-Simulink Converter2/1 -> Product/1, Bus Element Out/1  "I_PV_load"
  Product/1 -> Bus Element Out2/1
  connections:
  Grid/RConn1 -- Simscape Bus1/RConn1
  Resistor/LConn1 -- Current Sensor1/RConn2 -- Controlled Current Source1/LConn1
  Voltage Sensor1/RConn2 -- Simscape Bus1/LConn2 -- Resistor/RConn1 -- Controlled Current Source1/RConn2
  Simscape Bus1/LConn1 -- Voltage Sensor1/LConn1 -- Current Sensor1/LConn1
  PS-Simulink Converter4/LConn1 -- PS-Simulink Converter3/LConn1 -- Voltage Sensor1/RConn1
  Simulink-PS Converter1/RConn1 -- Controlled Current Source1/RConn1
  PS-Simulink Converter2/LConn1 -- Current Sensor1/RConn1

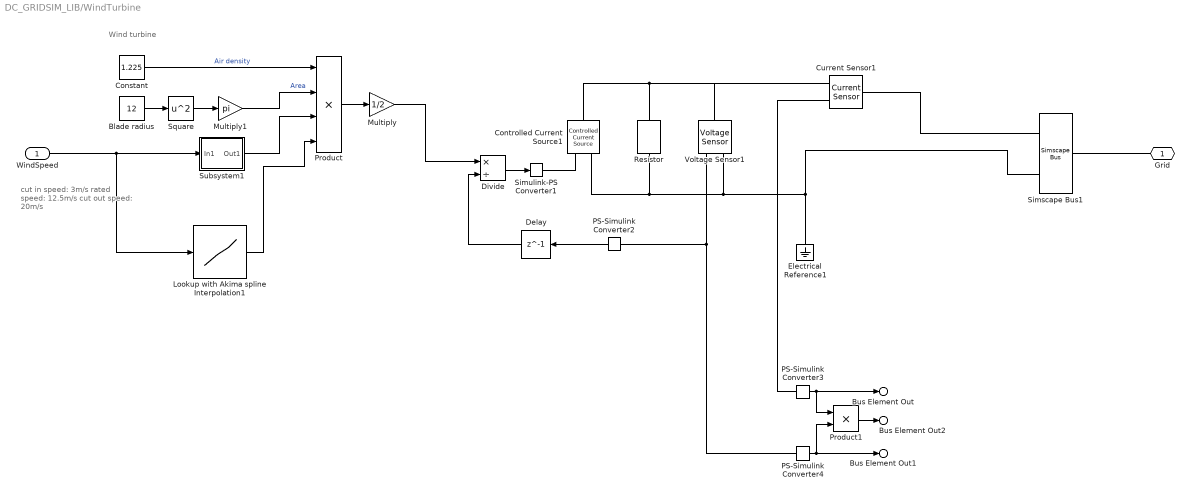
== system DC_GRIDSIM_LIB/WindTurbine ==
  note: cut in speed: 3m/s
      | rated speed: 12.5m/s
      | cut out speed: 20m/s
  note: Wind turbine
  WindSpeed : Inport
  Blade radius : Constant  Value=12
  Constant : Constant  Value=1.225
  Controlled Current Source1 : fl_lib/Electrical/Electrical Sources/Controlled Current Source
  Current Sensor1 : fl_lib/Electrical/Electrical Sensors/Current Sensor
  Delay : Delay  DelayLength=1  InitialCondition=MV
  Divide : Product  Inputs=*/
  Electrical Reference1 : fl_lib/Electrical/Electrical Elements/Electrical Reference
  Lookup with Akima spline Interpolation1 : Lookup_n-D  NumberOfTableDimensions=1  BreakpointsForDimension1=[0;1;2;3;3.5;4;4.5;5;5.5;6;6.5;7;7.5;8;8.5;9;9.5;10;10.5;11;11.5;12;13;14;15;16;17;18;19]  Table=[0;0;0;0.13;0.15;0.17;0.19;0.23;0.26;0.29;0.32;0.35;0.37;0.39;0.4;0.4;0.39;0.35;0.3;0.26;0.23;0.2;0;0;0;0;0;0;0]  InterpMethod=Akima spline  InternalRulePriority=Speed  OutDataTypeStr=double  RndMeth=Simplest
  Multiply : Gain  Gain=1/2
  Multiply1 : Gain  Gain=pi
  PS-Simulink Converter2 : nesl_utility/PS-Simulink Converter  PhysicalDomain=network_engine_domain  SubClassName=ps_output  LeftPortType=input  RightPortType=output  PseudoPeriodic=off  Frequencies=[]  VectorFormat=inherit  Unit=inherit  AffineConversion=off
  PS-Simulink Converter3 : nesl_utility/PS-Simulink Converter  PhysicalDomain=network_engine_domain  SubClassName=ps_output  LeftPortType=input  RightPortType=output  PseudoPeriodic=off  Frequencies=[]  VectorFormat=inherit  Unit=inherit  AffineConversion=off
  PS-Simulink Converter4 : nesl_utility/PS-Simulink Converter  PhysicalDomain=network_engine_domain  SubClassName=ps_output  LeftPortType=input  RightPortType=output  PseudoPeriodic=off  Frequencies=[]  VectorFormat=inherit  Unit=inherit  AffineConversion=off
  Product : Product  Inputs=4
  Product1 : Product
  Resistor : fl_lib/Electrical/Electrical Elements/Resistor  R=1e9 Ohm  i_specify=off  i_priority=None  i=0 A  i_nominal_specify=off  i_nominal_unit=A  i_nominal_value=1  v_specify=off  v_priority=None  v=0 V  v_nominal_specify=off  v_nominal_unit=V  v_nominal_value=1
  Simscape Bus1 : SimscapeBus  HierarchyStrings=High;Low
  Simulink-PS Converter1 : nesl_utility/Simulink-PS Converter  PhysicalDomain=network_engine_domain  SubClassName=ps_input  LeftPortType=input  RightPortType=output  PseudoPeriodic=off  Frequencies=[]  NoiseDistribution=none  NoiseParameters=[]  Unit=1  AffineConversion=off  FilteringAndDerivatives=provide  SimscapeFilterOrder=1  InputFilterTimeConstant=0.001  UdotUserProvided=0
  Square : Math  Operator=square
  Subsystem1 : Subsystem
      mask Display: disp('Vw^3');
  Voltage Sensor1 : fl_lib/Electrical/Electrical Sensors/Voltage Sensor
  Grid : PMIOPort  Side=Right
  Bus Element Out : Outport  PortName=Meas  Element=Current
  Bus Element Out1 : Outport  PortName=Meas  Element=Voltage
  Bus Element Out2 : Outport  PortName=Meas  Element=Power
  wires:
  Lookup with Akima spline Interpolation1/1 -> Product/4
  Multiply1/1 -> Product/2  "Area"
  Blade radius/1 -> Square/1
  Square/1 -> Multiply1/1
  Constant/1 -> Product/1  "Air density"
  WindSpeed/1 -> Lookup with Akima spline Interpolation1/1, Subsystem1/1(In1)
  Product/1 -> Multiply/1
  Subsystem1/1(Out1) -> Product/3
  Delay/1 -> Divide/2
  PS-Simulink Converter4/1 -> Product1/2, Bus Element Out1/1
  Divide/1 -> Simulink-PS Converter1/1
  PS-Simulink Converter3/1 -> Product1/1, Bus Element Out/1
  Multiply/1 -> Divide/1
  PS-Simulink Converter2/1 -> Delay/1
  Product1/1 -> Bus Element Out2/1
  connections:
  Grid/RConn1 -- Simscape Bus1/RConn1
  Controlled Current Source1/RConn2 -- Voltage Sensor1/RConn2 -- Simscape Bus1/LConn2 -- Electrical Reference1/LConn1 -- Resistor/RConn1
  Resistor/LConn1 -- Voltage Sensor1/LConn1 -- Current Sensor1/RConn2 -- Controlled Current Source1/LConn1
  PS-Simulink Converter4/LConn1 -- Voltage Sensor1/RConn1 -- PS-Simulink Converter2/LConn1
  PS-Simulink Converter3/LConn1 -- Current Sensor1/RConn1
  Simulink-PS Converter1/RConn1 -- Controlled Current Source1/RConn1
  Current Sensor1/LConn1 -- Simscape Bus1/LConn1

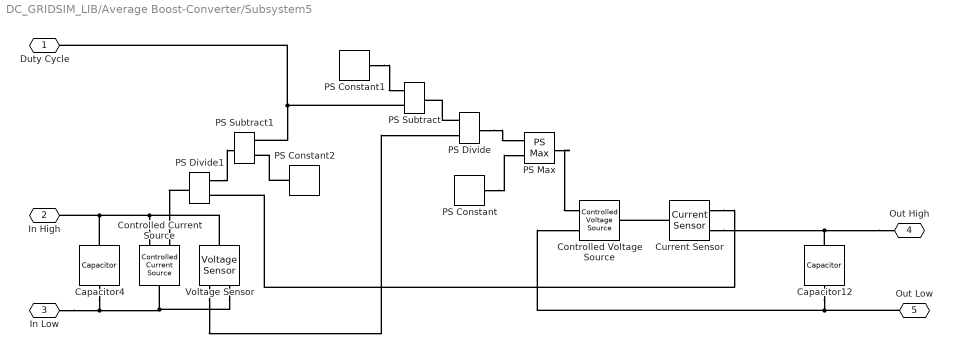
== system DC_GRIDSIM_LIB/Average Boost-Converter/Subsystem5 ==
  Capacitor12 : fl_lib/Electrical/Electrical Elements/Capacitor  c=C uF  r=1e-6 Ohm  g=0 1/Ohm  i_specify=off  i_priority=None  i=1 A  i_nominal_specify=off  i_nominal_unit=A  i_nominal_value=1  v_specify=off  v_priority=None  v=48 V  v_nominal_specify=off  v_nominal_unit=V  v_nominal_value=1  vc_specify=off  vc_priority=High  vc=48 V  vc_nominal_specify=off  vc_nominal_unit=V  vc_nominal_value=1
  Capacitor4 : fl_lib/Electrical/Electrical Elements/Capacitor  c=C uF  r=1e-6 Ohm  g=0 1/Ohm  i_specify=off  i_priority=None  i=1 A  i_nominal_specify=off  i_nominal_unit=A  i_nominal_value=1  v_specify=off  v_priority=None  v=48 V  v_nominal_specify=off  v_nominal_unit=V  v_nominal_value=1  vc_specify=off  vc_priority=High  vc=48 V  vc_nominal_specify=off  vc_nominal_unit=V  vc_nominal_value=1
  Controlled Current Source : fl_lib/Electrical/Electrical Sources/Controlled Current Source
  Controlled Voltage Source : fl_lib/Electrical/Electrical Sources/Controlled Voltage Source
  Current Sensor : fl_lib/Electrical/Electrical Sensors/Current Sensor
  PS Constant : fl_lib/Physical Signals/Sources/PS Constant  constant=1e-3 V
  PS Constant1 : fl_lib/Physical Signals/Sources/PS Constant  constant=1
  PS Constant2 : fl_lib/Physical Signals/Sources/PS Constant  constant=1
  PS Divide : fl_lib/Physical Signals/Functions/PS Divide
  PS Divide1 : fl_lib/Physical Signals/Functions/PS Divide
  PS Max : fl_lib/Physical Signals/Nonlinear Operators/PS Max
      settings: InternalSimscapePortConfiguration="{\"Bottom\":[],\"Left\":[{\"id\":\"I1\",\"label\":\"\",\"type\":\"input\"},{\"id\":\"I2\",\"label\":\"\",\"type\":\"input\"}],\"Right\":[{\"id\":\"O\",\"label\":\"\",\"type\":\"output\"}],\"Top\":[]}"
  PS Subtract : fl_lib/Physical Signals/Functions/PS Subtract
  PS Subtract1 : fl_lib/Physical Signals/Functions/PS Subtract
  Voltage Sensor : fl_lib/Electrical/Electrical Sensors/Voltage Sensor
  Duty Cycle : PMIOPort  Side=Left
  In High : PMIOPort  Port=2  Side=Left
  In Low : PMIOPort  Port=3  Side=Left
  Out High : PMIOPort  Port=4  Side=Right
  Out Low : PMIOPort  Port=5  Side=Right
  connections:
  In High/RConn1 -- Controlled Current Source/RConn2 -- Voltage Sensor/LConn1 -- Capacitor4/LConn1
  Capacitor12/RConn1 -- Out Low/RConn1 -- Controlled Voltage Source/RConn2
  Controlled Current Source/LConn1 -- Voltage Sensor/RConn2 -- In Low/RConn1 -- Capacitor4/RConn1
  Out High/RConn1 -- Current Sensor/RConn2 -- Capacitor12/LConn1
  Duty Cycle/RConn1 -- PS Subtract/LConn2 -- PS Subtract1/LConn2
  PS Divide1/LConn2 -- PS Subtract1/RConn1
  PS Divide/RConn1 -- PS Max/LConn1
  PS Constant2/RConn1 -- PS Subtract1/LConn1
  PS Constant1/RConn1 -- PS Subtract/LConn1
  PS Divide1/RConn1 -- Controlled Current Source/RConn1
  Voltage Sensor/RConn1 -- PS Divide/LConn1
  PS Divide/LConn2 -- PS Subtract/RConn1
  PS Max/RConn1 -- Controlled Voltage Source/RConn1
  Current Sensor/LConn1 -- Controlled Voltage Source/LConn1
  Current Sensor/RConn1 -- PS Divide1/LConn1
  PS Constant/RConn1 -- PS Max/LConn2
